simulink subsystem "AP5"  (R2019b)
settings: Solver=VariableStepAuto  StartTime=0.0  StopTime=10.0  RelTol=1e-3
model mask{sync_byte=71, msg_len=6}
  mask prompts: sync_byte "Byte value for detecting the start of a message."; msg_len "Fixed expected message length."
InitFcn:
  | %% DSPBuilder Start
  | alt_dspbuilder_update_model(bdroot)
  | %% DSPBuilder End
StartFcn:
  | %% DSPBuilder Start
  | alt_dspbuilder_hdlimport_prepare_for_simulation(bdroot)
  | %% DSPBuilder End
libraries: allblocks_alteradspbuilder2 x7
settings Model: Creator=vboxuser  LastModifiedBy=vboxuser

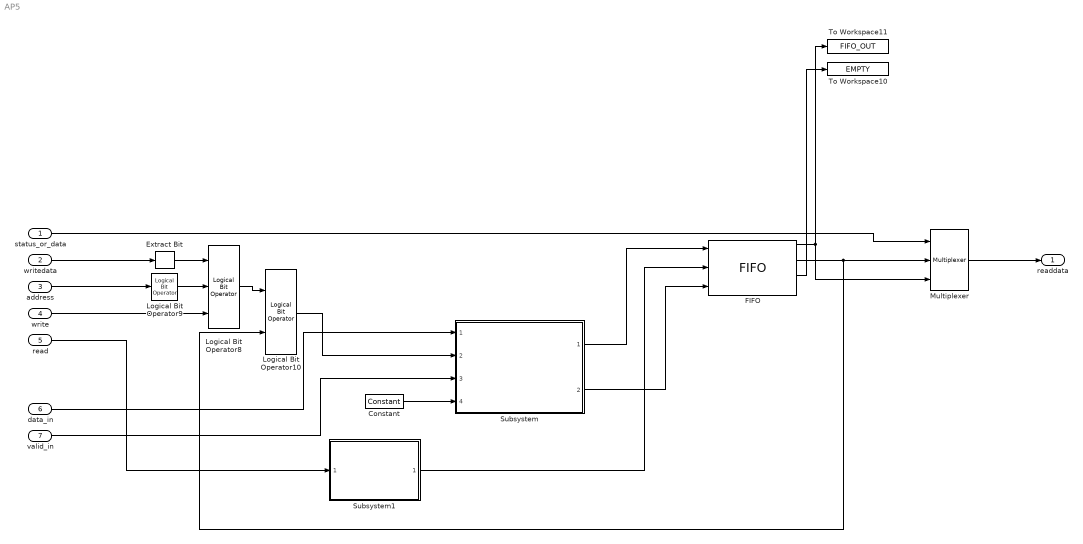
== system AP5 ==
  status_or_data : Inport
  writedata : Inport  Port=2
  address : Inport  Port=3
  write : Inport  Port=4
  read : Inport  Port=5
  data_in : Inport  Port=6
  valid_in : Inport  Port=7
  Constant : allblocks_alteradspbuilder2/Constant  mask_cst=sync_byte  BusType=Signed Integer  bwl=8  bwr=0  roundMode=Truncate  satMode=Wrap  SpecifyClock=off  allowFloatingPointOverride=on  logOutputs=off  logFile=C:\Users\vboxuser\Documents\MATLAB\serializer\system2\tb_AP5\AP5_Constant.fixedpointlog
  Extract Bit : allblocks_alteradspbuilder2/Extract Bit  BusType=Unsigned Integer  bwl=32  bwr=1  bitToSelect=0  pipeline_display=0
  FIFO : allblocks_alteradspbuilder2/FIFO  numwords=msg_len  BusType=Signed Integer  bwl=8  bwr=0  ram_type=AUTO  use_sclr=off  use_les_only=off  showahead_mode=off  allowFloatingPointOverride=on  logOutputs=off  logFile=C:\Users\vboxuser\Documents\MATLAB\serializer\system2\tb_AP5\AP5_FIFO%3A%3Aq.fixedpointlog,C:\Users\vboxuser\Documents\MATLAB\serializer\system2\tb_AP5\AP5_FIFO%3A%3Afull.fixedpointlog,C:\Users\vboxuser\Documents\MATLAB\serializer\system2\tb_AP5\AP5_FIFO%3A%3Aempty.fixedpointlog,C:\Users\vboxuser\Documents\MATLAB\serializer\system2\tb_AP5\AP5_FIFO%3A%3Ausedw.fixedpointlog,
  Logical Bit Operator10 : allblocks_alteradspbuilder2/Logical Bit Operator  LogicalOperator=OR  user_inputs=2  pipeline_display=0
  Logical Bit Operator8 : allblocks_alteradspbuilder2/Logical Bit Operator  LogicalOperator=AND  user_inputs=3  pipeline_display=0
  Logical Bit Operator9 : allblocks_alteradspbuilder2/Logical Bit Operator  LogicalOperator=NOT  user_inputs=2  pipeline_display=0
  Multiplexer : allblocks_alteradspbuilder2/Multiplexer  numInputs=2  pipeline=0  oneHot=off  pipeline_display=0  use_ena=off  use_aclr=off  allowFloatingPointOverride=on  logOutputs=off  logFile=C:\AP5_Multiplexer.fixedpointlog
  Subsystem : Subsystem  ReferencedSubsystem=decoder
  Subsystem1 : Subsystem  ReferencedSubsystem=Puls
  To Workspace10 : ToWorkspace  VariableName=EMPTY  SampleTime=-1
      settings: Save2DSignal=2-D array (concatenate along first dimension)
  To Workspace11 : ToWorkspace  VariableName=FIFO_OUT  SampleTime=-1
      settings: Save2DSignal=2-D array (concatenate along first dimension)
  readdata : Outport
  wires:
  Logical Bit Operator8/1 -> Logical Bit Operator10/1
  Subsystem/2 -> FIFO/3
  Subsystem1/1 -> FIFO/2
  FIFO/1 -> Multiplexer/3, To Workspace11/1
  Subsystem/1 -> FIFO/1
  FIFO/2 -> Multiplexer/2, Logical Bit Operator10/2
  data_in/1 -> Subsystem/1
  Multiplexer/1 -> readdata/1
  Logical Bit Operator10/1 -> Subsystem/2
  writedata/1 -> Extract Bit/1
  FIFO/3 -> To Workspace10/1
  Logical Bit Operator9/1 -> Logical Bit Operator8/2
  Extract Bit/1 -> Logical Bit Operator8/1
  read/1 -> Subsystem1/1
  valid_in/1 -> Subsystem/3
  status_or_data/1 -> Multiplexer/1
  write/1 -> Logical Bit Operator8/3
  address/1 -> Logical Bit Operator9/1
  Constant/1 -> Subsystem/4
